simulink model "closedloopPcontroller"  (R2016a)
settings: Solver=FixedStepAuto  StartTime=0.0  StopTime=50  RelTol=1e-3
undefined symbols (not defined in the file): closedloop, Motor, Subsystem
libraries: arduinolib x5, dspadpt3 x1
settings Model: SimulationMode=external  ExtModeTrigDuration=2  Creator=dell  LastModifiedBy=dell
settings OptimizationCC: OptimizeModelRefInitCode=on  LifeSpan=1  MaxStackSize=64
settings HardwareCC: ProdBitPerInt=16  ProdBitPerPointer=16  ProdLargestAtomicFloat=None  ProdWordSize=8  ProdHWDeviceType=Atmel->AVR
settings RTWCC: SystemTargetFile=ert.tlc  HardwareBoard=Arduino Mega 2560  TemplateMakefile=ert_default_tmf  GenerateReport=on  Toolchain=Arduino AVR v1.6.1  BuildConfiguration=Faster Runs  IncludeHyperlinkInReport=on  LaunchReport=on  GenerateTraceInfo=on  GenerateTraceReport=on  GenerateTraceReportSl=on  GenerateTraceReportSf=on  GenerateTraceReportEml=on
settings CodeAppCC: ForceParamTrailComments=on  IgnoreCustomStorageClasses=off  OperatorAnnotations=on  SimulinkDataObjDesc=on  SFDataObjDesc=on  MATLABFcnDesc=on  InsertBlockDesc=on  MATLABSourceComments=on
settings ERTTargetCC: SupportContinuousTime=on  SupportVariableSizeSignals=on

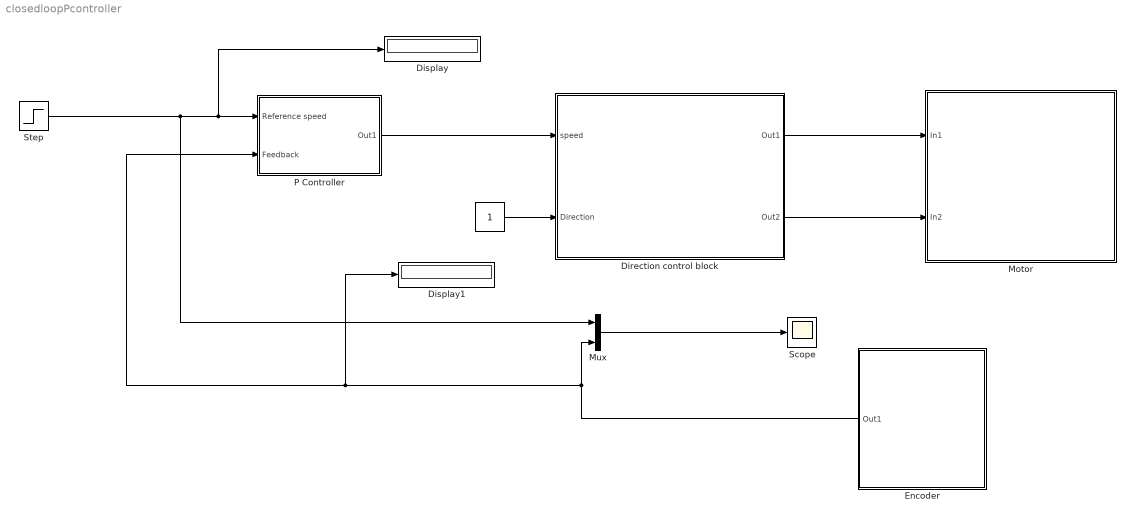
== system closedloopPcontroller ==
  " " : Constant
  Direction control block : Subsystem  AncestorBlock=closedloop/Subsystem
  Display : Display
  Display1 : Display
  "Encoder " : Subsystem
  Motor : Subsystem  AncestorBlock=closedloop/Motor
  Mux : Mux  Inputs=2
  P Controller : Subsystem
  Scope : Scope
  Step : Step  Time=5  After=185  SampleTime=0
  wires:
  Direction control block/1(Out1) -> Motor/1(In1)
  Direction control block/2(Out2) -> Motor/2(In2)
  Mux/1 -> Scope/1
  P Controller/1(Out1) -> Direction control block/1(speed)
  "Encoder "/1(Out1) -> Mux/2, Display1/1, P Controller/2(Feedback)
  " "/1 -> Direction control block/2(Direction)
  Step/1 -> Mux/1, Display/1, P Controller/1(Reference speed)

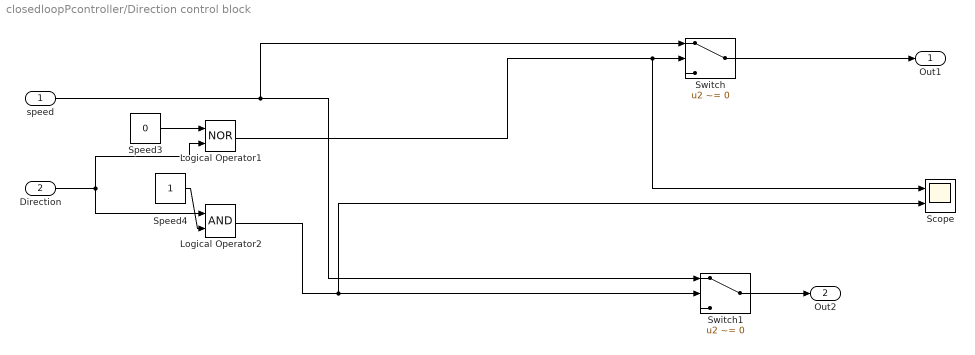
== system closedloopPcontroller/Direction control block ==
  speed : Inport
  Direction : Inport  Port=2
  Logical Operator1 : Logic  Operator=NOR  AllPortsSameDT=off  OutDataTypeStr=boolean
  Logical Operator2 : Logic  AllPortsSameDT=off  OutDataTypeStr=boolean
  Scope : Scope  NumInputPorts=2
  Speed3 : Constant  Value=0  OutMin=0  OutMax=100  OutDataTypeStr=single  SampleTime=0.001
  Speed4 : Constant  OutMin=0  OutMax=100  OutDataTypeStr=single  SampleTime=0.001
  Switch : Switch  Criteria=u2 ~= 0
  Switch1 : Switch  Criteria=u2 ~= 0
  Out1 : Outport
  Out2 : Outport  Port=2
  wires:
  Speed3/1 -> Logical Operator1/1
  speed/1 -> Switch/1, Switch1/1
  Switch1/1 -> Out2/1
  Switch/1 -> Out1/1
  Direction/1 -> Logical Operator2/1, Logical Operator1/2
  Logical Operator2/1 -> Scope/2, Switch1/2
  Speed4/1 -> Logical Operator2/2
  Logical Operator1/1 -> Scope/1, Switch/2

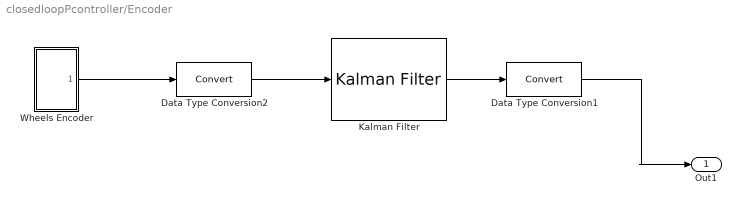
== system closedloopPcontroller/Encoder  ==
  " Wheels Encoder" : Subsystem  AncestorBlock=closedloop/Right Wheels Encoder
  Data Type Conversion1 : DataTypeConversion
  Data Type Conversion2 : DataTypeConversion
  Kalman Filter : dspadpt3/Kalman Filter  num_targets=1  sourceEnable=Always  isReset=on  X=zeros([1])  P=10*eye(1)  A=[1]  sourceMeasure=Specify via Dialog  H=[1]  Q=0.0005*eye(1)  R=eye(1)  isOutputEstMeasure=on  isOutputEstState=off  isOutputEstError=off  isOutputPrdMeasure=off  isOutputPrdState=off  isOutputPrdError=off
  Out1 : Outport
  wires:
  " Wheels Encoder"/1(Encoder) -> Data Type Conversion2/1
  Data Type Conversion2/1 -> Kalman Filter/1
  Kalman Filter/1 -> Data Type Conversion1/1
  Data Type Conversion1/1 -> Out1/1

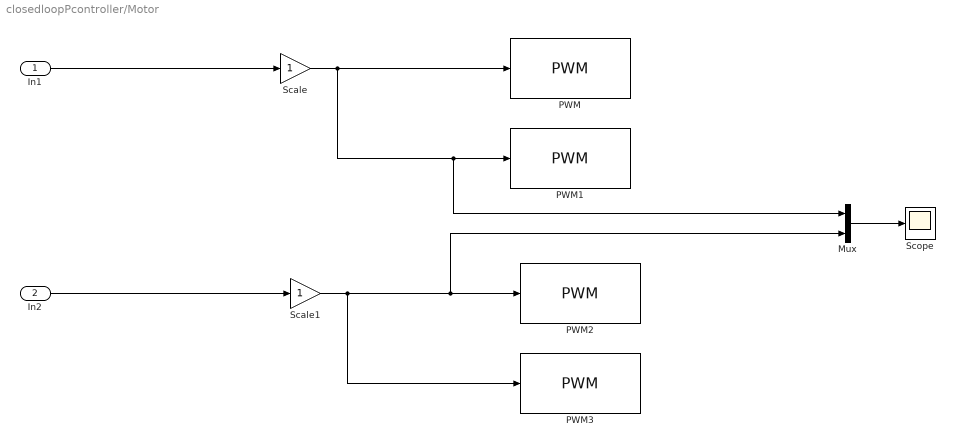
== system closedloopPcontroller/Motor ==
  In1 : Inport
  In2 : Inport  Port=2
  Mux : Mux  Inputs=2
  PWM : arduinolib/PWM  pinNumber=5  blockPlatform=arduino
  PWM1 : arduinolib/PWM  pinNumber=11  blockPlatform=arduino
  PWM2 : arduinolib/PWM  pinNumber=4  blockPlatform=arduino
  PWM3 : arduinolib/PWM  pinNumber=6  blockPlatform=arduino
  Scale : Gain
  Scale1 : Gain
  Scope : Scope
  wires:
  In1/1 -> Scale/1
  Scale/1 -> PWM/1, Mux/1, PWM1/1
  In2/1 -> Scale1/1
  Mux/1 -> Scope/1
  Scale1/1 -> Mux/2, PWM2/1, PWM3/1

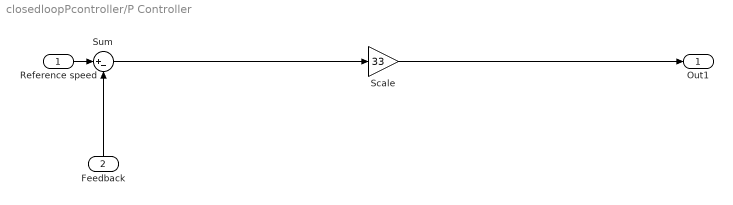
== system closedloopPcontroller/P Controller ==
  Reference speed : Inport
  Feedback : Inport  Port=2
  Scale : Gain  Gain=33
  Sum : Sum  Inputs=|+-
  Out1 : Outport
  wires:
  Reference speed/1 -> Sum/1
  Feedback/1 -> Sum/2
  Sum/1 -> Scale/1
  Scale/1 -> Out1/1

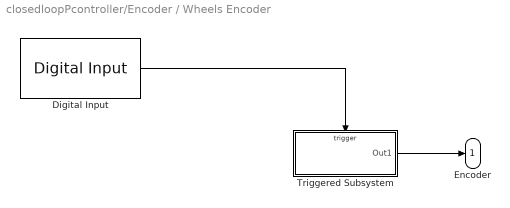
== system closedloopPcontroller/Encoder / Wheels Encoder ==
  Digital Input : arduinolib/Digital Input  pinNumber=2  sampleTime=0.001  blockPlatform=arduino
  Triggered Subsystem : Subsystem  TreatAsAtomicUnit=on
  Encoder : Outport
  wires:
  Digital Input/1 -> Triggered Subsystem/Trigger
  Triggered Subsystem/1(Out1) -> Encoder/1

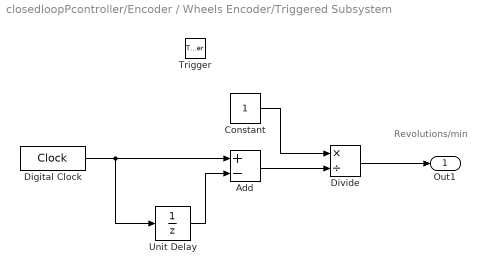
== system closedloopPcontroller/Encoder / Wheels Encoder/Triggered Subsystem ==
  note: Revolutions/min
  Trigger : TriggerPort  VariantControl=Variant
  Add : Sum  Inputs=+-
  Constant : Constant
  Digital Clock : DigitalClock  SampleTime=-1
  Divide : Product  Inputs=*/  OutDataTypeStr=int32
  Unit Delay : UnitDelay  SampleTime=-1
  Out1 : Outport
  wires:
  Constant/1 -> Divide/1
  Divide/1 -> Out1/1
  Add/1 -> Divide/2
  Unit Delay/1 -> Add/2
  Digital Clock/1 -> Unit Delay/1, Add/1
